simulink library "slrtnpcinverterlib"  (R2022b)
settings: Solver=VariableStepAuto  StartTime=0.0  StopTime=10.0  RelTol=1e-3
libraries: simulink x39, slrthdlutillib x6, $bdroot x3, hdlsllib x1
settings Model: Creator=chrisz  LastModifiedBy=chrisz
settings ModelReferenceCC: EnableRefExpFcnMdlSchedulingChecks=on

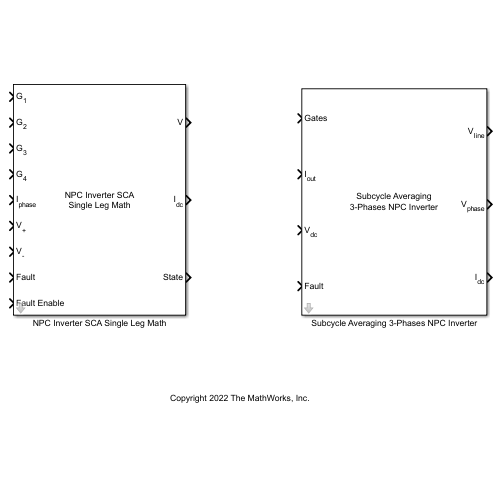
[thumbnail: Simulink's stored preview of the top-level diagram]
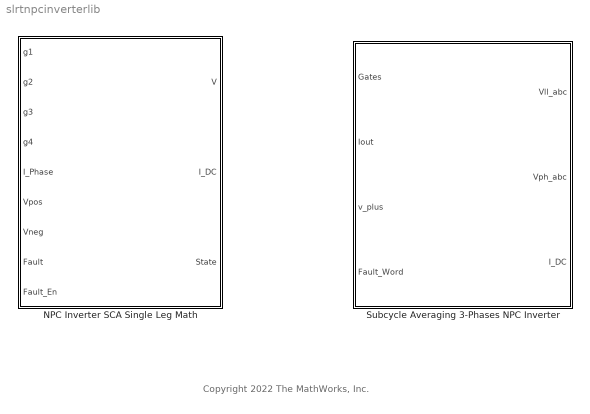
== system slrtnpcinverterlib ==
  note: Copyright 2022 The MathWorks, Inc.
  NPC Inverter SCA Single Leg Math : Subsystem  mask(NPC Inverter SCA Single Leg Math){rIGBT=0.1, vfIGBT=0.8, rDiode=0.2, vfDiode=0.6, rSnub=1e5, ts_Model=1e-6, ts_FPGA=5e-9}
      mask prompts: rIGBT "IGBT Resistance (Ohms):"; vfIGBT "IGBT Forward Voltage (V):"; rDiode "Diode Resistance (Ohms):"; vfDiode "Diode Forward Voltage (V):"; rSnub "Snubber resistance (Ohms):"; ts_Model "Model Time Step (s):"; ts_FPGA "FPGA Time Step (s):"
      mask help: This block implements the algorithm for a single leg of subcycle averaging NPC inverter. This model simulates FPGA clock level operations and is not suited for desktop simulation other than for validating the real-time model is accurate. It should primarily be used when generating HDL for real-time systems. Use standard blocks for desktop simulation.
      mask DialogControl Container6 Prompt: Simulation Parameters
      mask Display:
      | disp('NPC Inverter SCA\nSingle Leg Math');
      | 
      | port_label('input', 1, 'G_1','texmode','on');
      | port_label('input', 2, 'G_2','texmode','on');
      | port_label('input', 3, 'G_3','texmode','on');
      | port_label('input', 4, 'G_4','texmode','on');
      | port_label('input', 5, 'I_p_h_a_s_e','texmode','on');
      | port_label('input', 6, 'V_+','texmode','on');
      | port_label('input', 7, 'V_-','texmode','on');
      | port_label('input', 8, 'Fault');
      | port_label('input', 9, 'Fault Enable');
      | port_label('output', 1, 'V');
      | port_label('output', 2, 'I_d_c','texmode','on');
      | port_label('output', 3, 'State');
  Subcycle Averaging 3-Phases NPC Inverter : Subsystem  mask(Subcycle Averaging 3-Phases NPC Inverter){rIGBT=0.1, vfIGBT=0.8, rDiode=0.2, vfDiode=0.6, rSnub=1e5, ts_Model=1e-6, ts_FPGA=5e-9}
      mask prompts: rIGBT "IGBT Resistance (Ohms):"; vfIGBT "IGBT Forward Voltage (V):"; rDiode "Diode Resistance (Ohms):"; vfDiode "Diode Forward Voltage (V):"; rSnub "Snubber resistance (Ohms):"; ts_Model "Model Time Step (s):"; ts_FPGA "FPGA Time Step (s):"
      mask help:
      | HDL compatible implementation of subcycle averaging 3-phases NPC inverter. This model simulates FPGA clock level operations and is not suited for desktop simulation other than for validating the real-time model is accurate. It should primarily be used when generating HDL for real-time systems. Use standard blocks for desktop simulation.
      |
      | Model time step should be 1/10 of switching frequency to capture accurate switching waveforms. FPGA time step should be the fastest time step you can run your HIL FPGA at.
      mask DialogControl Container3 Prompt: Simulation Parameters
      mask Display:
      | disp('Subcycle Averaging\n3-Phases NPC Inverter')
      | port_label('input',1,'Gates');
      | port_label('input',2,'I_o_u_t','texmode','on');
      | port_label('input',3,'V_d_c','texmode','on');
      | port_label('input',4,'Fault');
      | 
      | port_label('output',1,'V_l_i_n_e','texmode','on');
      | port_label('output',2,'V_p_h_a_s_e','texmode','on');
      | port_label('output',3,'I_d_c','texmode','on');

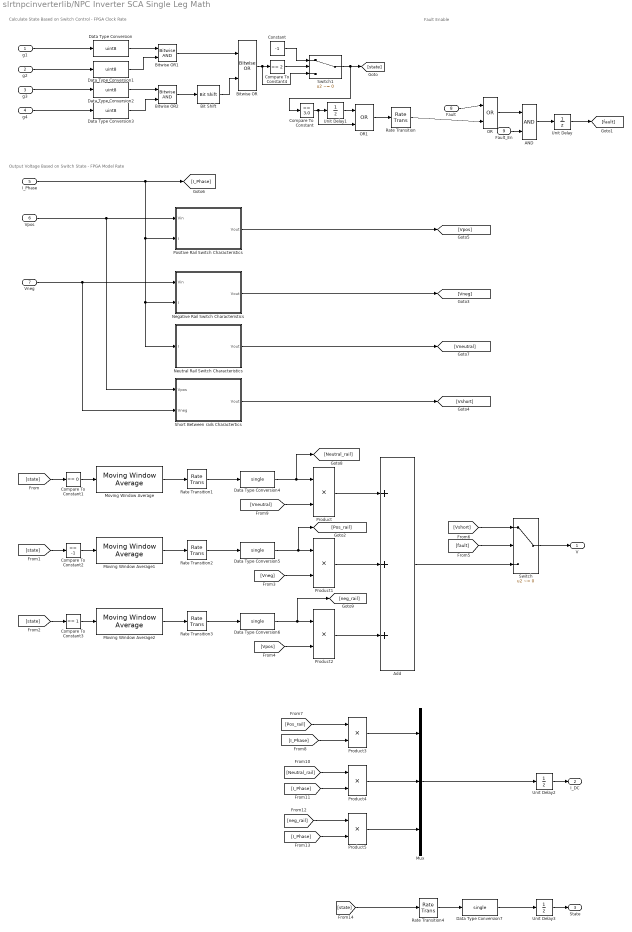
== system slrtnpcinverterlib/NPC Inverter SCA Single Leg Math ==
  note: Output Voltage Based on Switch State - FPGA Model Rate
  note: Fault Enable
  note: Calculate State Based on Switch Control - FPGA Clock Rate
  g1 : Inport
  g2 : Inport  Port=2
  g3 : Inport  Port=3
  g4 : Inport  Port=4
  I_Phase : Inport  Port=5
  Vpos : Inport  Port=6
  Vneg : Inport  Port=7
  Fault : Inport  Port=8
  Fault_En : Inport  Port=9
  AND : Logic  IconShape=distinctive  AllPortsSameDT=off  OutDataTypeStr=boolean
  Add : Sum  Inputs=+++
  Bit Shift : hdlsllib/Logic and Bit Operations/Bit Shift  mode=Shift Left Logical  N=1
  Bitwise OR : simulink/Logic and Bit Operations/Bitwise Operator  logicop=OR  UseBitMask=off  NumInputPorts=2  BitMask=bin2dec('11011001')  BitMaskRealWorld=Stored Integer
  Bitwise OR1 : simulink/Logic and Bit Operations/Bitwise Operator  logicop=AND  UseBitMask=off  NumInputPorts=2  BitMask=bin2dec('11011001')  BitMaskRealWorld=Stored Integer
  Bitwise OR2 : simulink/Logic and Bit Operations/Bitwise Operator  logicop=AND  UseBitMask=off  NumInputPorts=2  BitMask=bin2dec('11011001')  BitMaskRealWorld=Stored Integer
  Compare To Constant : simulink/Logic and Bit Operations/Compare To Constant  relop===  const=3.0  OutDataTypeStr=boolean
  Compare To Constant1 : simulink/Logic and Bit Operations/Compare To Constant  relop===  const=0  OutDataTypeStr=boolean
  Compare To Constant2 : simulink/Logic and Bit Operations/Compare To Constant  relop===  const=-1  OutDataTypeStr=boolean
  Compare To Constant3 : simulink/Logic and Bit Operations/Compare To Constant  relop===  const=1  OutDataTypeStr=boolean
  Compare To Constant4 : simulink/Logic and Bit Operations/Compare To Constant  relop===  const=2  OutDataTypeStr=boolean
  Constant : Constant  Value=-1  OutDataTypeStr=int8  SampleTime=-1
  Data Type Conversion{,1..3} (4 alike) : DataTypeConversion  OutDataTypeStr=uint8  SaturateOnIntegerOverflow=off  RndMeth=Floor
  Data Type Conversion{4..7} (4 alike) : DataTypeConversion  OutDataTypeStr=single  SaturateOnIntegerOverflow=off  RndMeth=Floor
  Moving Window Average : slrthdlutillib/Moving Window Average  sample_time=ts_FPGA  window_size=ts_Model
  Moving Window Average1 : slrthdlutillib/Moving Window Average  sample_time=ts_FPGA  window_size=ts_Model
  Moving Window Average2 : slrthdlutillib/Moving Window Average  sample_time=ts_FPGA  window_size=ts_Model
  Mux : Mux  Inputs=3
  Negative Rail Switch Characteristics : Subsystem
  Neutral Rail Switch Characteristics : Subsystem
  OR : Logic  Operator=OR  IconShape=distinctive  AllPortsSameDT=off  OutDataTypeStr=boolean
  OR1 : Logic  Operator=OR  IconShape=distinctive  AllPortsSameDT=off  OutDataTypeStr=boolean
  Positive Rail Switch Characteristics : Subsystem
  Product{,1..5} (6 alike) : Product
  Rate Transition{,1..4} (5 alike) : RateTransition  OutPortSampleTime=ts_Model
  Short Between rails Charactertics : Subsystem
  Switch : Switch  Criteria=u2 ~= 0  SaturateOnIntegerOverflow=off  InputSameDT=off
  Switch1 : Switch  Criteria=u2 ~= 0  OutDataTypeStr=int8  SaturateOnIntegerOverflow=off  InputSameDT=off
  Unit Delay{,1..3} (4 alike) : UnitDelay  SampleTime=-1  HasFrameUpgradeWarning=on
  V : Outport
  I_DC : Outport  Port=2
  State : Outport  Port=3
  wires:
  Fault/1 -> OR/1
  Data Type Conversion/1 -> Bitwise OR1/1
  Bitwise OR/1 -> Switch1/3, Compare To Constant4/1
  Data Type Conversion3/1 -> Bitwise OR2/2
  Data Type Conversion1/1 -> Bitwise OR1/2
  Data Type Conversion2/1 -> Bitwise OR2/1
  [state] -> Compare To Constant1/1
  g1/1 -> Data Type Conversion/1
  g2/1 -> Data Type Conversion1/1
  g3/1 -> Data Type Conversion2/1
  g4/1 -> Data Type Conversion3/1
  OR/1 -> AND/1
  Fault_En/1 -> AND/2
  AND/1 -> Unit Delay/1
  Unit Delay/1 -> [fault]
  Compare To Constant/1 -> OR1/2, Unit Delay1/1
  Unit Delay1/1 -> OR1/1
  Rate Transition/1 -> OR/2
  OR1/1 -> Rate Transition/1
  Vneg/1 -> Short Between rails Charactertics/2(Vneg), Negative Rail Switch Characteristics/1(Vin)
  Vpos/1 -> Short Between rails Charactertics/1(Vpos), Positive Rail Switch Characteristics/1(Vin)
  Positive Rail Switch Characteristics/1(Vout) -> [Vpos]
  Negative Rail Switch Characteristics/1(Vout) -> [Vneg]
  Short Between rails Charactertics/1(Vout) -> [Vshort]
  [state] -> Compare To Constant2/1
  [state] -> Compare To Constant3/1
  Compare To Constant1/1 -> Moving Window Average/1
  Compare To Constant2/1 -> Moving Window Average1/1
  Compare To Constant3/1 -> Moving Window Average2/1
  Moving Window Average/1 -> Rate Transition1/1
  Moving Window Average1/1 -> Rate Transition2/1
  Moving Window Average2/1 -> Rate Transition3/1
  Rate Transition1/1 -> Data Type Conversion4/1
  Rate Transition2/1 -> Data Type Conversion5/1
  Rate Transition3/1 -> Data Type Conversion6/1
  Data Type Conversion4/1 -> [Neutral_rail], Product/1
  [Vneutral] -> Product/2
  Data Type Conversion5/1 -> [Pos_rail], Product1/1
  [Vneg] -> Product1/2
  Data Type Conversion6/1 -> [neg_rail], Product2/1
  [Vpos] -> Product2/2
  Product/1 -> Add/1
  Product1/1 -> Add/2
  Product2/1 -> Add/3
  [fault] -> Switch/2
  [Vshort] -> Switch/1
  Add/1 -> Switch/3
  Switch/1 -> V/1
  [Pos_rail] -> Product3/1
  I_Phase/1 -> [I_Phase], Positive Rail Switch Characteristics/2(I), Neutral Rail Switch Characteristics/1(I), Negative Rail Switch Characteristics/2(I)
  [I_Phase] -> Product3/2
  Unit Delay2/1 -> I_DC/1
  Neutral Rail Switch Characteristics/1(Vout) -> [Vneutral]
  [Neutral_rail] -> Product4/1
  [I_Phase] -> Product4/2
  [neg_rail] -> Product5/1
  [I_Phase] -> Product5/2
  Product3/1 -> Mux/1
  Product4/1 -> Mux/2
  Product5/1 -> Mux/3
  Mux/1 -> Unit Delay2/1
  Bitwise OR2/1 -> Bit Shift/1
  Bit Shift/1 -> Bitwise OR/2
  Bitwise OR1/1 -> Bitwise OR/1
  Compare To Constant4/1 -> Switch1/2
  Switch1/1 -> Compare To Constant/1, [state]
  Constant/1 -> Switch1/1
  Data Type Conversion7/1 -> Unit Delay3/1
  Unit Delay3/1 -> State/1
  [state] -> Rate Transition4/1
  Rate Transition4/1 -> Data Type Conversion7/1

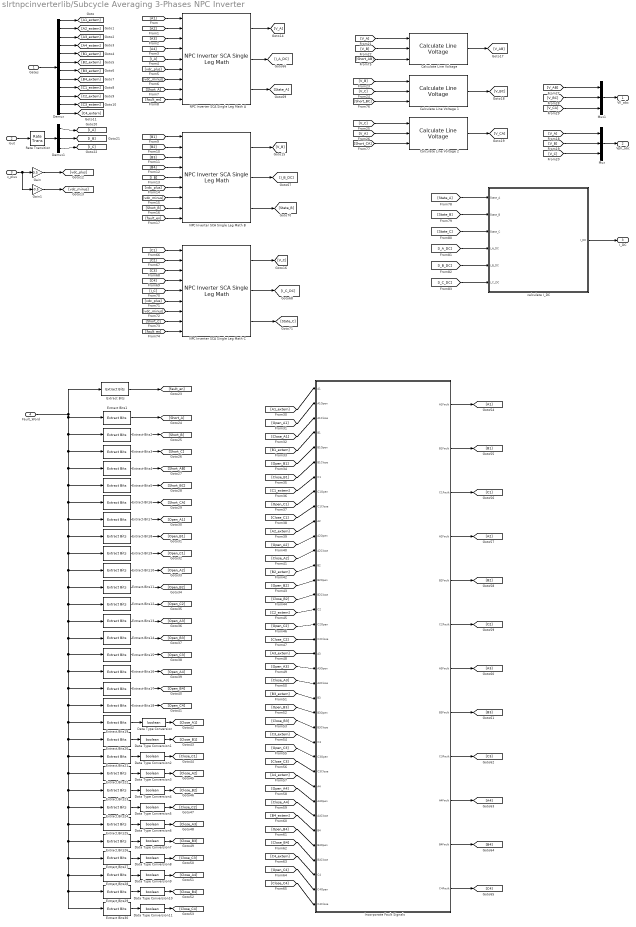
== system slrtnpcinverterlib/Subcycle Averaging 3-Phases NPC Inverter ==
  Gates : Inport
  Iout : Inport  Port=2
  v_plus : Inport  Port=3
  Fault_Word : Inport  Port=4
  "Calculate Line Voltage " : slrthdlutillib/Calculate Line Voltage 
  Calculate Line Voltage 1 : slrthdlutillib/Calculate Line Voltage 
  Calculate Line Voltage 2 : slrthdlutillib/Calculate Line Voltage 
  Data Type Conversion{,1..11} (12 alike) : DataTypeConversion  OutDataTypeStr=boolean  SaturateOnIntegerOverflow=off  RndMeth=Floor
  Demux : Demux  Outputs=12
  Demux1 : Demux  Outputs=3
  Extract Bits : simulink/Logic and Bit Operations/Extract Bits  bitsToExtract=Range of bits  numBits=8  bitIdxRange=31  outScalingMode=Treat bit field as an integer
  Extract Bits1 : simulink/Logic and Bit Operations/Extract Bits  bitsToExtract=Range of bits  numBits=8  bitIdxRange=0  outScalingMode=Treat bit field as an integer
  Extract Bits10 : simulink/Logic and Bit Operations/Extract Bits  bitsToExtract=Range of bits  numBits=8  bitIdxRange=9  outScalingMode=Treat bit field as an integer
  Extract Bits11 : simulink/Logic and Bit Operations/Extract Bits  bitsToExtract=Range of bits  numBits=8  bitIdxRange=10  outScalingMode=Treat bit field as an integer
  Extract Bits12 : simulink/Logic and Bit Operations/Extract Bits  bitsToExtract=Range of bits  numBits=8  bitIdxRange=11  outScalingMode=Treat bit field as an integer
  Extract Bits13 : simulink/Logic and Bit Operations/Extract Bits  bitsToExtract=Range of bits  numBits=8  bitIdxRange=12  outScalingMode=Treat bit field as an integer
  Extract Bits14 : simulink/Logic and Bit Operations/Extract Bits  bitsToExtract=Range of bits  numBits=8  bitIdxRange=13  outScalingMode=Treat bit field as an integer
  Extract Bits15 : simulink/Logic and Bit Operations/Extract Bits  bitsToExtract=Range of bits  numBits=8  bitIdxRange=14  outScalingMode=Treat bit field as an integer
  Extract Bits16 : simulink/Logic and Bit Operations/Extract Bits  bitsToExtract=Range of bits  numBits=8  bitIdxRange=15  outScalingMode=Treat bit field as an integer
  Extract Bits17 : simulink/Logic and Bit Operations/Extract Bits  bitsToExtract=Range of bits  numBits=8  bitIdxRange=16  outScalingMode=Treat bit field as an integer
  Extract Bits18 : simulink/Logic and Bit Operations/Extract Bits  bitsToExtract=Range of bits  numBits=8  bitIdxRange=17  outScalingMode=Treat bit field as an integer
  Extract Bits19 : simulink/Logic and Bit Operations/Extract Bits  bitsToExtract=Range of bits  numBits=8  bitIdxRange=18  outScalingMode=Treat bit field as an integer
  Extract Bits2 : simulink/Logic and Bit Operations/Extract Bits  bitsToExtract=Range of bits  numBits=8  bitIdxRange=1  outScalingMode=Treat bit field as an integer
  Extract Bits20 : simulink/Logic and Bit Operations/Extract Bits  bitsToExtract=Range of bits  numBits=8  bitIdxRange=19  outScalingMode=Treat bit field as an integer
  Extract Bits21 : simulink/Logic and Bit Operations/Extract Bits  bitsToExtract=Range of bits  numBits=8  bitIdxRange=20  outScalingMode=Treat bit field as an integer
  Extract Bits22 : simulink/Logic and Bit Operations/Extract Bits  bitsToExtract=Range of bits  numBits=8  bitIdxRange=21  outScalingMode=Treat bit field as an integer
  Extract Bits23 : simulink/Logic and Bit Operations/Extract Bits  bitsToExtract=Range of bits  numBits=8  bitIdxRange=22  outScalingMode=Treat bit field as an integer
  Extract Bits24 : simulink/Logic and Bit Operations/Extract Bits  bitsToExtract=Range of bits  numBits=8  bitIdxRange=23  outScalingMode=Treat bit field as an integer
  Extract Bits25 : simulink/Logic and Bit Operations/Extract Bits  bitsToExtract=Range of bits  numBits=8  bitIdxRange=24  outScalingMode=Treat bit field as an integer
  Extract Bits26 : simulink/Logic and Bit Operations/Extract Bits  bitsToExtract=Range of bits  numBits=8  bitIdxRange=25  outScalingMode=Treat bit field as an integer
  Extract Bits27 : simulink/Logic and Bit Operations/Extract Bits  bitsToExtract=Range of bits  numBits=8  bitIdxRange=26  outScalingMode=Treat bit field as an integer
  Extract Bits28 : simulink/Logic and Bit Operations/Extract Bits  bitsToExtract=Range of bits  numBits=8  bitIdxRange=27  outScalingMode=Treat bit field as an integer
  Extract Bits29 : simulink/Logic and Bit Operations/Extract Bits  bitsToExtract=Range of bits  numBits=8  bitIdxRange=28  outScalingMode=Treat bit field as an integer
  Extract Bits3 : simulink/Logic and Bit Operations/Extract Bits  bitsToExtract=Range of bits  numBits=8  bitIdxRange=2  outScalingMode=Treat bit field as an integer
  Extract Bits30 : simulink/Logic and Bit Operations/Extract Bits  bitsToExtract=Range of bits  numBits=8  bitIdxRange=29  outScalingMode=Treat bit field as an integer
  Extract Bits4 : simulink/Logic and Bit Operations/Extract Bits  bitsToExtract=Range of bits  numBits=8  bitIdxRange=3  outScalingMode=Treat bit field as an integer
  Extract Bits5 : simulink/Logic and Bit Operations/Extract Bits  bitsToExtract=Range of bits  numBits=8  bitIdxRange=4  outScalingMode=Treat bit field as an integer
  Extract Bits6 : simulink/Logic and Bit Operations/Extract Bits  bitsToExtract=Range of bits  numBits=8  bitIdxRange=5  outScalingMode=Treat bit field as an integer
  Extract Bits7 : simulink/Logic and Bit Operations/Extract Bits  bitsToExtract=Range of bits  numBits=8  bitIdxRange=6  outScalingMode=Treat bit field as an integer
  Extract Bits8 : simulink/Logic and Bit Operations/Extract Bits  bitsToExtract=Range of bits  numBits=8  bitIdxRange=7  outScalingMode=Treat bit field as an integer
  Extract Bits9 : simulink/Logic and Bit Operations/Extract Bits  bitsToExtract=Range of bits  numBits=8  bitIdxRange=8  outScalingMode=Treat bit field as an integer
  Gain : Gain  Gain=0.5
  Gain1 : Gain  Gain=-0.5
  Incorporate Fault Signals : Subsystem
  Mux : Mux  Inputs=3
  Mux1 : Mux  Inputs=3
  NPC Inverter SCA Single Leg Math A : $bdroot/NPC Inverter SCA Single Leg Math  rIGBT=rIGBT  vfIGBT=vfIGBT  rDiode=rDiode  vfDiode=vfDiode  rSnub=rSnub  ts_Model=ts_Model  ts_FPGA=ts_FPGA
  NPC Inverter SCA Single Leg Math B : $bdroot/NPC Inverter SCA Single Leg Math  rIGBT=rIGBT  vfIGBT=vfIGBT  rDiode=rDiode  vfDiode=vfDiode  rSnub=rSnub  ts_Model=ts_Model  ts_FPGA=ts_FPGA
  NPC Inverter SCA Single Leg Math C : $bdroot/NPC Inverter SCA Single Leg Math  rIGBT=rIGBT  vfIGBT=vfIGBT  rDiode=rDiode  vfDiode=vfDiode  rSnub=rSnub  ts_Model=ts_Model  ts_FPGA=ts_FPGA
  Rate Transition : RateTransition  OutPortSampleTime=ts_Model
  calculate I_DC : Subsystem
  Vll_abc : Outport
  Vph_abc : Outport  Port=2
  I_DC : Outport  Port=3
  wires:
  Gates/1 -> Demux/1
  Demux/1 -> [A1_extern]
  Demux/2 -> [A2_extern]
  Demux/3 -> [A3_extern]
  Demux/4 -> [A4_extern]
  Demux/5 -> [B1_extern]
  Demux/6 -> [B2_extern]
  Demux/7 -> [B3_extern]
  Demux/8 -> [B4_extern]
  Demux/9 -> [C1_extern]
  Demux/10 -> [C2_extern]
  Demux/11 -> [C3_extern]
  Demux/12 -> [C4_extern]
  Gain1/1 -> [vdc_minus]
  NPC Inverter SCA Single Leg Math A/1 -> [V_A]
  NPC Inverter SCA Single Leg Math B/1 -> [V_B]
  NPC Inverter SCA Single Leg Math C/1 -> [V_C]
  Mux/1 -> Vph_abc/1
  [V_A] -> Mux/1
  [V_B] -> Mux/2
  [V_C] -> Mux/3
  [V_A] -> "Calculate Line Voltage "/1
  [V_B] -> "Calculate Line Voltage "/2
  "Calculate Line Voltage "/1 -> [V_AB]
  [V_C] -> Calculate Line Voltage 1/2
  [V_B] -> Calculate Line Voltage 1/1
  Calculate Line Voltage 1/1 -> [V_BC]
  [V_A] -> Calculate Line Voltage 2/2
  [V_C] -> Calculate Line Voltage 2/1
  Calculate Line Voltage 2/1 -> [V_CA]
  Mux1/1 -> Vll_abc/1
  [V_AB] -> Mux1/1
  [V_BC] -> Mux1/2
  [V_CA] -> Mux1/3
  Demux1/1 -> [I_A]
  Demux1/2 -> [I_B]
  Demux1/3 -> [I_C]
  Fault_Word/1 -> Extract Bits/1, Extract Bits7/1, Extract Bits8/1, Extract Bits9/1, Extract Bits10/1, Extract Bits11/1, Extract Bits12/1, Extract Bits13/1, Extract Bits14/1, Extract Bits16/1, Extract Bits17/1, Extract Bits19/1, Extract Bits20/1, Extract Bits21/1, Extract Bits22/1, Extract Bits23/1, Extract Bits24/1, Extract Bits25/1, Extract Bits26/1, Extract Bits27/1, Extract Bits28/1, Extract Bits29/1, Extract Bits30/1, Extract Bits18/1, Extract Bits15/1, Extract Bits6/1, Extract Bits5/1, Extract Bits4/1, Extract Bits3/1, Extract Bits2/1, Extract Bits1/1
  Extract Bits/1 -> [fault_en]
  Extract Bits1/1 -> [Short_A]
  Extract Bits2/1 -> [Short_B]
  Extract Bits3/1 -> [Short_C]
  Extract Bits4/1 -> [Short_AB]
  Extract Bits5/1 -> [Short_BC]
  Extract Bits6/1 -> [Short_CA]
  Extract Bits7/1 -> [Open_A1]
  Extract Bits8/1 -> [Open_B1]
  Extract Bits9/1 -> [Open_C1]
  Extract Bits10/1 -> [Open_A2]
  Extract Bits12/1 -> [Open_C2]
  Extract Bits11/1 -> [Open_B2]
  Extract Bits13/1 -> [Open_A3]
  Extract Bits15/1 -> [Open_C3]
  Extract Bits14/1 -> [Open_B3]
  Extract Bits18/1 -> [Open_C4]
  Extract Bits17/1 -> [Open_B4]
  Extract Bits16/1 -> [Open_A4]
  [A1_extern] -> Incorporate Fault Signals/1(A1)
  [Open_A1] -> Incorporate Fault Signals/2(A1Open)
  [Close_A1] -> Incorporate Fault Signals/3(A1Close)
  [Close_B1] -> Incorporate Fault Signals/6(B1Close)
  [Open_B1] -> Incorporate Fault Signals/5(B1Open)
  [B1_extern] -> Incorporate Fault Signals/4(B1)
  [C1_extern] -> Incorporate Fault Signals/7(C1)
  [Open_C1] -> Incorporate Fault Signals/8(C1Open)
  [Close_C1] -> Incorporate Fault Signals/9(C1Close)
  [A2_extern] -> Incorporate Fault Signals/10(A2)
  [Open_A2] -> Incorporate Fault Signals/11(A2Open)
  [Close_A2] -> Incorporate Fault Signals/12(A2Close)
  [Close_B2] -> Incorporate Fault Signals/15(B2Close)
  [Open_B2] -> Incorporate Fault Signals/14(B2Open)
  [B2_extern] -> Incorporate Fault Signals/13(B2)
  [C2_extern] -> Incorporate Fault Signals/16(C2)
  [Open_C2] -> Incorporate Fault Signals/17(C2Open)
  [Close_C2] -> Incorporate Fault Signals/18(C2Close)
  [Close_A3] -> Incorporate Fault Signals/21(A3Close)
  [Open_A3] -> Incorporate Fault Signals/20(A3Open)
  [A3_extern] -> Incorporate Fault Signals/19(A3)
  [Close_B3] -> Incorporate Fault Signals/24(B3Close)
  [Open_B3] -> Incorporate Fault Signals/23(B3Open)
  [B3_extern] -> Incorporate Fault Signals/22(B3)
  [Close_C3] -> Incorporate Fault Signals/27(C3Close)
  [Open_C3] -> Incorporate Fault Signals/26(C3Open)
  [C3_extern] -> Incorporate Fault Signals/25(C3)
  [Close_A4] -> Incorporate Fault Signals/30(A4Close)
  [Open_A4] -> Incorporate Fault Signals/29(A4Open)
  [A4_extern] -> Incorporate Fault Signals/28(A4)
  [Close_B4] -> Incorporate Fault Signals/33(B4Close)
  [Open_B4] -> Incorporate Fault Signals/32(B4Open)
  [B4_extern] -> Incorporate Fault Signals/31(B4)
  [Close_C4] -> Incorporate Fault Signals/36(C4Close)
  [Open_C4] -> Incorporate Fault Signals/35(C4Open)
  [C4_extern] -> Incorporate Fault Signals/34(C4)
  Incorporate Fault Signals/1(A1Fault) -> [A1]
  Incorporate Fault Signals/2(B1Fault) -> [B1]
  Incorporate Fault Signals/3(C1Fault) -> [C1]
  Incorporate Fault Signals/4(A2Fault) -> [A2]
  Incorporate Fault Signals/5(B2Fault) -> [B2]
  Incorporate Fault Signals/6(C2Fault) -> [C2]
  Incorporate Fault Signals/7(A3Fault) -> [A3]
  Incorporate Fault Signals/8(B3Fault) -> [B3]
  Incorporate Fault Signals/9(C3Fault) -> [C3]
  Incorporate Fault Signals/10(A4Fault) -> [A4]
  Incorporate Fault Signals/11(B4Fault) -> [B4]
  Incorporate Fault Signals/12(C4Fault) -> [C4]
  [A1] -> NPC Inverter SCA Single Leg Math A/1
  [A2] -> NPC Inverter SCA Single Leg Math A/2
  [A3] -> NPC Inverter SCA Single Leg Math A/3
  [A4] -> NPC Inverter SCA Single Leg Math A/4
  [I_A] -> NPC Inverter SCA Single Leg Math A/5
  [vdc_plus] -> NPC Inverter SCA Single Leg Math A/6
  [vdc_minus] -> NPC Inverter SCA Single Leg Math A/7
  [Short_A] -> NPC Inverter SCA Single Leg Math A/8
  [fault_en] -> NPC Inverter SCA Single Leg Math A/9
  [B1] -> NPC Inverter SCA Single Leg Math B/1
  [B2] -> NPC Inverter SCA Single Leg Math B/2
  [B3] -> NPC Inverter SCA Single Leg Math B/3
  [B4] -> NPC Inverter SCA Single Leg Math B/4
  [I_B] -> NPC Inverter SCA Single Leg Math B/5
  [vdc_plus] -> NPC Inverter SCA Single Leg Math B/6
  [vdc_minus] -> NPC Inverter SCA Single Leg Math B/7
  [Short_B] -> NPC Inverter SCA Single Leg Math B/8
  [fault_en] -> NPC Inverter SCA Single Leg Math B/9
  [C1] -> NPC Inverter SCA Single Leg Math C/1
  [C2] -> NPC Inverter SCA Single Leg Math C/2
  [C3] -> NPC Inverter SCA Single Leg Math C/3
  [C4] -> NPC Inverter SCA Single Leg Math C/4
  [I_C] -> NPC Inverter SCA Single Leg Math C/5
  [vdc_plus] -> NPC Inverter SCA Single Leg Math C/6
  [vdc_minus] -> NPC Inverter SCA Single Leg Math C/7
  [Short_C] -> NPC Inverter SCA Single Leg Math C/8
  [fault_en] -> NPC Inverter SCA Single Leg Math C/9
  NPC Inverter SCA Single Leg Math A/2 -> [I_A_DC]
  NPC Inverter SCA Single Leg Math B/2 -> [I_B_DC]
  NPC Inverter SCA Single Leg Math C/2 -> [I_C_DC]
  [Short_AB] -> "Calculate Line Voltage "/3
  [Short_BC] -> Calculate Line Voltage 1/3
  [Short_CA] -> Calculate Line Voltage 2/3
  Data Type Conversion/1 -> [Close_A1]
  Extract Bits19/1 -> Data Type Conversion/1
  Data Type Conversion1/1 -> [Close_B1]
  Extract Bits20/1 -> Data Type Conversion1/1
  Extract Bits21/1 -> Data Type Conversion2/1
  Data Type Conversion2/1 -> [Close_C1]
  Extract Bits22/1 -> Data Type Conversion3/1
  Data Type Conversion3/1 -> [Close_A2]
  Extract Bits23/1 -> Data Type Conversion4/1
  Data Type Conversion4/1 -> [Close_B2]
  Extract Bits24/1 -> Data Type Conversion5/1
  Data Type Conversion5/1 -> [Close_C2]
  Extract Bits25/1 -> Data Type Conversion6/1
  Extract Bits26/1 -> Data Type Conversion7/1
  Extract Bits27/1 -> Data Type Conversion8/1
  Extract Bits28/1 -> Data Type Conversion9/1
  Extract Bits29/1 -> Data Type Conversion10/1
  Data Type Conversion6/1 -> [Close_A3]
  Data Type Conversion7/1 -> [Close_B3]
  Data Type Conversion8/1 -> [Close_C3]
  Data Type Conversion9/1 -> [Close_A4]
  Data Type Conversion10/1 -> [Close_B4]
  Extract Bits30/1 -> Data Type Conversion11/1
  Data Type Conversion11/1 -> [Close_C4]
  Iout/1 -> Rate Transition/1
  Rate Transition/1 -> Demux1/1
  v_plus/1 -> Gain1/1, Gain/1
  Gain/1 -> [vdc_plus]
  NPC Inverter SCA Single Leg Math A/3 -> [State_A]
  NPC Inverter SCA Single Leg Math B/3 -> [State_B]
  NPC Inverter SCA Single Leg Math C/3 -> [State_C]
  calculate I_DC/1(I_DC) -> I_DC/1
  [State_A] -> calculate I_DC/1(State_A)
  [State_B] -> calculate I_DC/2(State_B)
  [State_C] -> calculate I_DC/3(State_C)
  [I_A_DC] -> calculate I_DC/4(I_A_DC)
  [I_B_DC] -> calculate I_DC/5(I_B_DC)
  [I_C_DC] -> calculate I_DC/6(I_C_DC)

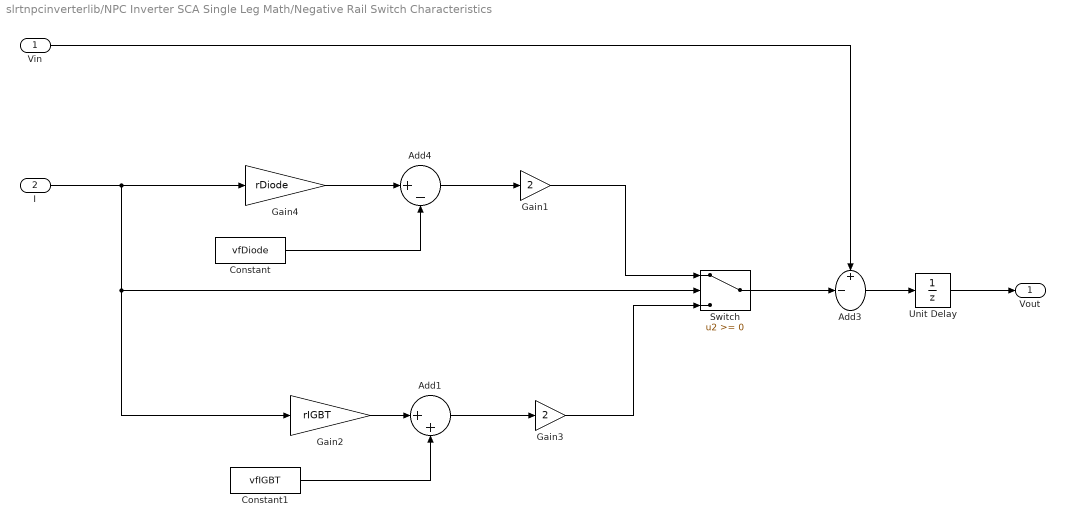
== system slrtnpcinverterlib/NPC Inverter SCA Single Leg Math/Negative Rail Switch Characteristics ==
  Vin : Inport
  I : Inport  Port=2
  Add1 : Sum  Inputs=|++
  Add3 : Sum  Inputs=+-|
  Add4 : Sum  Inputs=|+-
  Constant : Constant  Value=vfDiode  OutDataTypeStr=single  SampleTime=ts_Model
  Constant1 : Constant  Value=vfIGBT  OutDataTypeStr=single  SampleTime=ts_Model
  Gain1 : Gain  Gain=2
  Gain2 : Gain  Gain=rIGBT
  Gain3 : Gain  Gain=2
  Gain4 : Gain  Gain=rDiode
  Switch : Switch  SaturateOnIntegerOverflow=off  InputSameDT=off
  Unit Delay : UnitDelay  SampleTime=-1  HasFrameUpgradeWarning=on
  Vout : Outport
  wires:
  I/1 -> Gain2/1, Switch/2, Gain4/1
  Unit Delay/1 -> Vout/1
  Vin/1 -> Add3/1
  Add1/1 -> Gain3/1
  Constant1/1 -> Add1/2
  Gain2/1 -> Add1/1
  Gain3/1 -> Switch/3
  Gain4/1 -> Add4/1
  Constant/1 -> Add4/2
  Add4/1 -> Gain1/1
  Add3/1 -> Unit Delay/1
  Switch/1 -> Add3/2
  Gain1/1 -> Switch/1

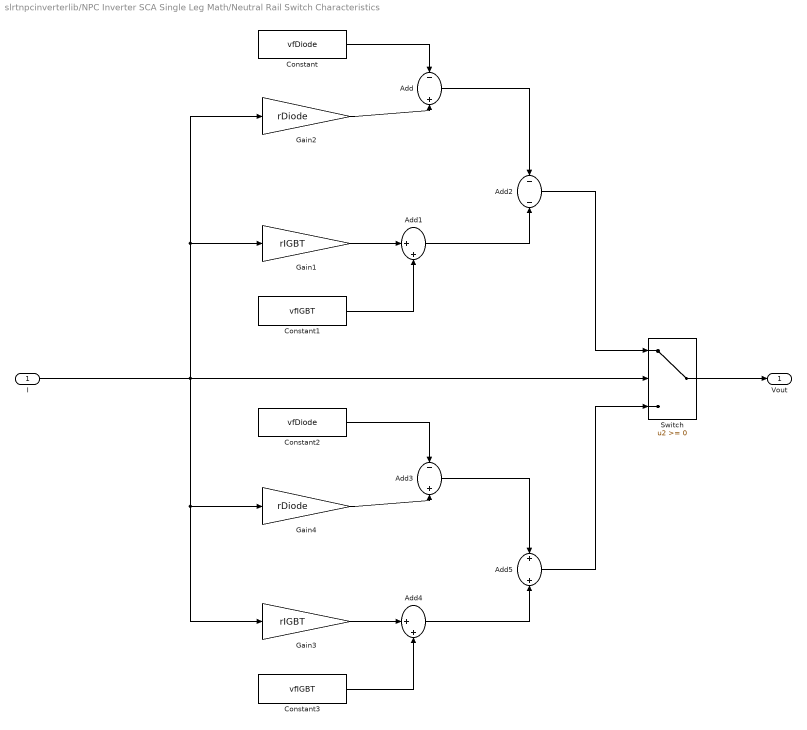
== system slrtnpcinverterlib/NPC Inverter SCA Single Leg Math/Neutral Rail Switch Characteristics ==
  I : Inport
  Add : Sum  Inputs=-+
  Add1 : Sum  Inputs=|++
  Add2 : Sum  Inputs=--
  Add3 : Sum  Inputs=-+
  Add4 : Sum  Inputs=|++
  Add5 : Sum
  Constant : Constant  Value=vfDiode  OutDataTypeStr=single  SampleTime=ts_Model
  Constant1 : Constant  Value=vfIGBT  OutDataTypeStr=single  SampleTime=ts_Model
  Constant2 : Constant  Value=vfDiode  OutDataTypeStr=single  SampleTime=ts_Model
  Constant3 : Constant  Value=vfIGBT  OutDataTypeStr=single  SampleTime=ts_Model
  Gain1 : Gain  Gain=rIGBT
  Gain2 : Gain  Gain=rDiode
  Gain3 : Gain  Gain=rIGBT
  Gain4 : Gain  Gain=rDiode
  Switch : Switch  SaturateOnIntegerOverflow=off  InputSameDT=off
  Vout : Outport
  wires:
  Gain1/1 -> Add1/1
  Constant1/1 -> Add1/2
  Add1/1 -> Add2/2
  Add5/1 -> Switch/3
  Add2/1 -> Switch/1
  Switch/1 -> Vout/1
  I/1 -> Gain4/1, Gain3/1, Gain2/1, Gain1/1, Switch/2
  Gain3/1 -> Add4/1
  Add4/1 -> Add5/2
  Constant3/1 -> Add4/2
  Gain2/1 -> Add/2
  Constant/1 -> Add/1
  Add/1 -> Add2/1
  Gain4/1 -> Add3/2
  Constant2/1 -> Add3/1
  Add3/1 -> Add5/1

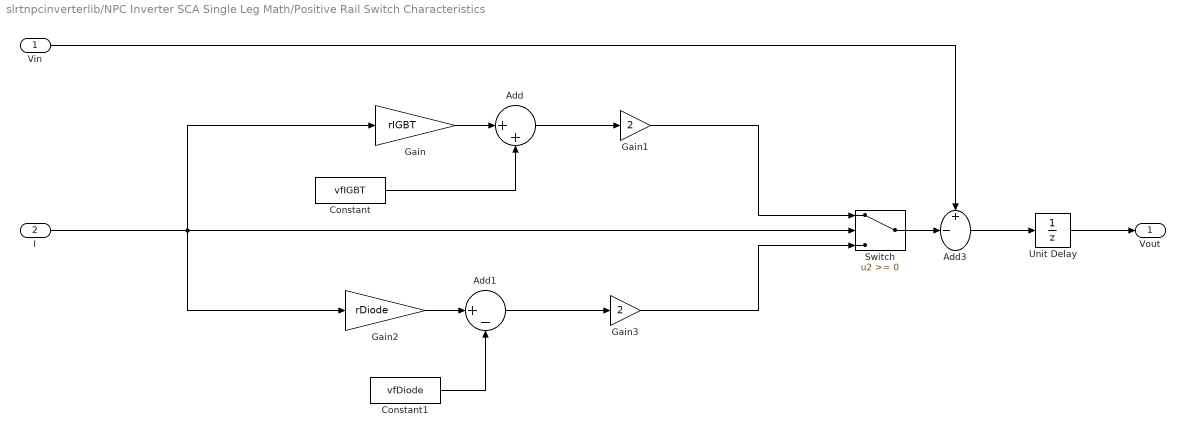
== system slrtnpcinverterlib/NPC Inverter SCA Single Leg Math/Positive Rail Switch Characteristics ==
  Vin : Inport
  I : Inport  Port=2
  Add : Sum  Inputs=|++
  Add1 : Sum  Inputs=|+-
  Add3 : Sum  Inputs=+-|
  Constant : Constant  Value=vfIGBT  OutDataTypeStr=single  SampleTime=ts_Model
  Constant1 : Constant  Value=vfDiode  OutDataTypeStr=single  SampleTime=ts_Model
  Gain : Gain  Gain=rIGBT
  Gain1 : Gain  Gain=2
  Gain2 : Gain  Gain=rDiode
  Gain3 : Gain  Gain=2
  Switch : Switch  SaturateOnIntegerOverflow=off  InputSameDT=off
  Unit Delay : UnitDelay  SampleTime=-1  HasFrameUpgradeWarning=on
  Vout : Outport
  wires:
  I/1 -> Gain2/1, Switch/2, Gain/1
  Gain/1 -> Add/1
  Constant/1 -> Add/2
  Add/1 -> Gain1/1
  Unit Delay/1 -> Vout/1
  Vin/1 -> Add3/1
  Gain3/1 -> Switch/3
  Gain2/1 -> Add1/1
  Add1/1 -> Gain3/1
  Constant1/1 -> Add1/2
  Add3/1 -> Unit Delay/1
  Switch/1 -> Add3/2
  Gain1/1 -> Switch/1

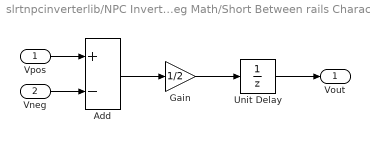
== system slrtnpcinverterlib/NPC Inverter SCA Single Leg Math/Short Between rails Charactertics ==
  Vpos : Inport
  Vneg : Inport  Port=2
  Add : Sum  Inputs=+-
  Gain : Gain  Gain=1/2
  Unit Delay : UnitDelay  SampleTime=-1  HasFrameUpgradeWarning=on
  Vout : Outport
  wires:
  Vpos/1 -> Add/1
  Vneg/1 -> Add/2
  Add/1 -> Gain/1
  Gain/1 -> Unit Delay/1
  Unit Delay/1 -> Vout/1

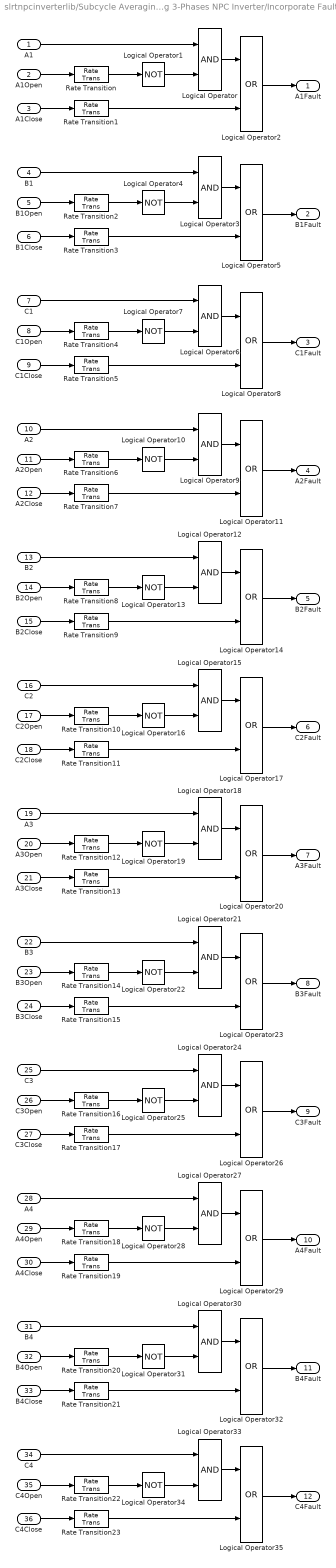
== system slrtnpcinverterlib/Subcycle Averaging 3-Phases NPC Inverter/Incorporate Fault Signals ==
  A1 : Inport
  A1Open : Inport  Port=2
  A1Close : Inport  Port=3
  B1 : Inport  Port=4
  B1Open : Inport  Port=5
  B1Close : Inport  Port=6
  C1 : Inport  Port=7
  C1Open : Inport  Port=8
  C1Close : Inport  Port=9
  A2 : Inport  Port=10
  A2Open : Inport  Port=11
  A2Close : Inport  Port=12
  B2 : Inport  Port=13
  B2Open : Inport  Port=14
  B2Close : Inport  Port=15
  C2 : Inport  Port=16
  C2Open : Inport  Port=17
  C2Close : Inport  Port=18
  A3 : Inport  Port=19
  A3Open : Inport  Port=20
  A3Close : Inport  Port=21
  B3 : Inport  Port=22
  B3Open : Inport  Port=23
  B3Close : Inport  Port=24
  C3 : Inport  Port=25
  C3Open : Inport  Port=26
  C3Close : Inport  Port=27
  A4 : Inport  Port=28
  A4Open : Inport  Port=29
  A4Close : Inport  Port=30
  B4 : Inport  Port=31
  B4Open : Inport  Port=32
  B4Close : Inport  Port=33
  C4 : Inport  Port=34
  C4Open : Inport  Port=35
  C4Close : Inport  Port=36
  Logical Operator{,3,6,9,12,15,18,21,24,27,30,33} (12 alike) : Logic  AllPortsSameDT=off  OutDataTypeStr=boolean
  Logical Operator{1,4,7,10,13,16,19,22,25,28,31,34} (12 alike) : Logic  Operator=NOT  AllPortsSameDT=off  OutDataTypeStr=boolean
  Logical Operator{2,5,8,11,14,17,20,23,26,29,32,35} (12 alike) : Logic  Operator=OR  AllPortsSameDT=off  OutDataTypeStr=boolean
  Rate Transition{,1..23} (24 alike) : RateTransition
  A1Fault : Outport
  B1Fault : Outport  Port=2
  C1Fault : Outport  Port=3
  A2Fault : Outport  Port=4
  B2Fault : Outport  Port=5
  C2Fault : Outport  Port=6
  A3Fault : Outport  Port=7
  B3Fault : Outport  Port=8
  C3Fault : Outport  Port=9
  A4Fault : Outport  Port=10
  B4Fault : Outport  Port=11
  C4Fault : Outport  Port=12
  wires:
  A1Open/1 -> Rate Transition/1
  A1Close/1 -> Rate Transition1/1
  Rate Transition/1 -> Logical Operator1/1
  Logical Operator1/1 -> Logical Operator/2
  A1/1 -> Logical Operator/1
  Logical Operator/1 -> Logical Operator2/1
  Rate Transition1/1 -> Logical Operator2/2
  Logical Operator2/1 -> A1Fault/1
  Rate Transition3/1 -> Logical Operator5/2
  B1Close/1 -> Rate Transition3/1
  Logical Operator4/1 -> Logical Operator3/2
  Rate Transition2/1 -> Logical Operator4/1
  B1/1 -> Logical Operator3/1
  Logical Operator5/1 -> B1Fault/1
  Logical Operator3/1 -> Logical Operator5/1
  B1Open/1 -> Rate Transition2/1
  Rate Transition5/1 -> Logical Operator8/2
  C1Close/1 -> Rate Transition5/1
  Logical Operator7/1 -> Logical Operator6/2
  Rate Transition4/1 -> Logical Operator7/1
  C1/1 -> Logical Operator6/1
  Logical Operator8/1 -> C1Fault/1
  Logical Operator6/1 -> Logical Operator8/1
  C1Open/1 -> Rate Transition4/1
  Rate Transition7/1 -> Logical Operator11/2
  A2Close/1 -> Rate Transition7/1
  Logical Operator10/1 -> Logical Operator9/2
  Rate Transition6/1 -> Logical Operator10/1
  Logical Operator15/1 -> Logical Operator17/1
  Rate Transition10/1 -> Logical Operator16/1
  C2/1 -> Logical Operator15/1
  Logical Operator16/1 -> Logical Operator15/2
  Logical Operator17/1 -> C2Fault/1
  Rate Transition11/1 -> Logical Operator17/2
  Rate Transition9/1 -> Logical Operator14/2
  A2/1 -> Logical Operator9/1
  Logical Operator11/1 -> A2Fault/1
  B2/1 -> Logical Operator12/1
  Logical Operator12/1 -> Logical Operator14/1
  C2Close/1 -> Rate Transition11/1
  C2Open/1 -> Rate Transition10/1
  B2Close/1 -> Rate Transition9/1
  Logical Operator13/1 -> Logical Operator12/2
  Logical Operator14/1 -> B2Fault/1
  B2Open/1 -> Rate Transition8/1
  Rate Transition8/1 -> Logical Operator13/1
  Logical Operator9/1 -> Logical Operator11/1
  A2Open/1 -> Rate Transition6/1
  Rate Transition13/1 -> Logical Operator20/2
  A3Close/1 -> Rate Transition13/1
  Logical Operator19/1 -> Logical Operator18/2
  Rate Transition12/1 -> Logical Operator19/1
  Logical Operator24/1 -> Logical Operator26/1
  Rate Transition16/1 -> Logical Operator25/1
  C3/1 -> Logical Operator24/1
  Logical Operator25/1 -> Logical Operator24/2
  Logical Operator26/1 -> C3Fault/1
  Rate Transition17/1 -> Logical Operator26/2
  Rate Transition15/1 -> Logical Operator23/2
  A3/1 -> Logical Operator18/1
  Logical Operator20/1 -> A3Fault/1
  B3/1 -> Logical Operator21/1
  Logical Operator21/1 -> Logical Operator23/1
  C3Close/1 -> Rate Transition17/1
  C3Open/1 -> Rate Transition16/1
  B3Close/1 -> Rate Transition15/1
  Logical Operator22/1 -> Logical Operator21/2
  Logical Operator23/1 -> B3Fault/1
  B3Open/1 -> Rate Transition14/1
  Rate Transition14/1 -> Logical Operator22/1
  Logical Operator18/1 -> Logical Operator20/1
  A3Open/1 -> Rate Transition12/1
  Rate Transition19/1 -> Logical Operator29/2
  A4Close/1 -> Rate Transition19/1
  Logical Operator28/1 -> Logical Operator27/2
  Rate Transition18/1 -> Logical Operator28/1
  Logical Operator33/1 -> Logical Operator35/1
  Rate Transition22/1 -> Logical Operator34/1
  C4/1 -> Logical Operator33/1
  Logical Operator34/1 -> Logical Operator33/2
  Logical Operator35/1 -> C4Fault/1
  Rate Transition23/1 -> Logical Operator35/2
  Rate Transition21/1 -> Logical Operator32/2
  A4/1 -> Logical Operator27/1
  Logical Operator29/1 -> A4Fault/1
  B4/1 -> Logical Operator30/1
  Logical Operator30/1 -> Logical Operator32/1
  C4Close/1 -> Rate Transition23/1
  C4Open/1 -> Rate Transition22/1
  B4Close/1 -> Rate Transition21/1
  Logical Operator31/1 -> Logical Operator30/2
  Logical Operator32/1 -> B4Fault/1
  B4Open/1 -> Rate Transition20/1
  Rate Transition20/1 -> Logical Operator31/1
  Logical Operator27/1 -> Logical Operator29/1
  A4Open/1 -> Rate Transition18/1

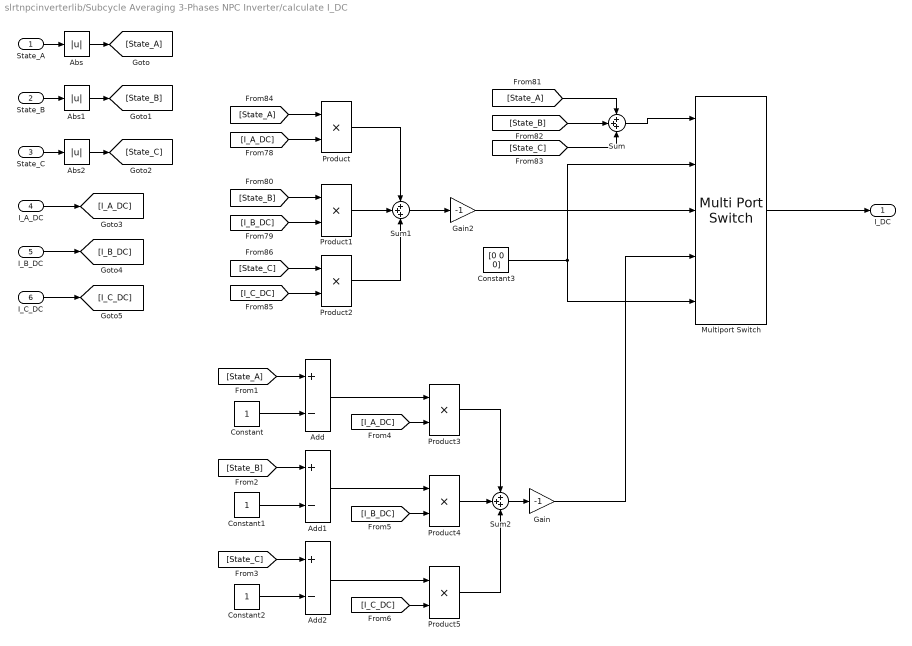
== system slrtnpcinverterlib/Subcycle Averaging 3-Phases NPC Inverter/calculate I_DC ==
  State_A : Inport
  State_B : Inport  Port=2
  State_C : Inport  Port=3
  I_A_DC : Inport  Port=4
  I_B_DC : Inport  Port=5
  I_C_DC : Inport  Port=6
  Abs : Abs  SaturateOnIntegerOverflow=off
  Abs1 : Abs  SaturateOnIntegerOverflow=off
  Abs2 : Abs  SaturateOnIntegerOverflow=off
  Add : Sum  Inputs=+-
  Add1 : Sum  Inputs=+-
  Add2 : Sum  Inputs=+-
  Constant : Constant  OutDataTypeStr=single  SampleTime=ts_Model
  Constant1 : Constant  OutDataTypeStr=single  SampleTime=ts_Model
  Constant2 : Constant  OutDataTypeStr=single  SampleTime=ts_Model
  Constant3 : Constant  Value=[0 0 0]  OutDataTypeStr=single  SampleTime=ts_Model
  Gain : Gain  Gain=-1
  Gain2 : Gain  Gain=-1
  Multiport Switch : MultiPortSwitch  DataPortOrder=Zero-based contiguous  Inputs=4  zeroidx=on  SaturateOnIntegerOverflow=off  InputSameDT=off
  Product{,1..5} (6 alike) : Product
  Sum : Sum  Inputs=+++
  Sum1 : Sum  Inputs=+++
  Sum2 : Sum  Inputs=+++
  I_DC : Outport
  wires:
  Product/1 -> Sum1/1
  [State_A] -> Product/1
  [I_A_DC] -> Product/2
  [State_B] -> Product1/1
  [I_C_DC] -> Product2/2
  Sum1/1 -> Gain2/1
  [I_B_DC] -> Product1/2
  [State_C] -> Product2/1
  Multiport Switch/1 -> I_DC/1
  [State_C] -> Sum/3
  Product1/1 -> Sum1/2
  [State_A] -> Sum/1
  Gain2/1 -> Multiport Switch/3
  [State_B] -> Sum/2
  Product2/1 -> Sum1/3
  Sum/1 -> Multiport Switch/1
  I_A_DC/1 -> [I_A_DC]
  I_B_DC/1 -> [I_B_DC]
  I_C_DC/1 -> [I_C_DC]
  [State_A] -> Add/1
  Constant/1 -> Add/2
  [State_B] -> Add1/1
  Constant1/1 -> Add1/2
  [State_C] -> Add2/1
  Constant2/1 -> Add2/2
  Add/1 -> Product3/1
  [I_A_DC] -> Product3/2
  [I_B_DC] -> Product4/2
  Add1/1 -> Product4/1
  [I_C_DC] -> Product5/2
  Add2/1 -> Product5/1
  Product3/1 -> Sum2/1
  Product4/1 -> Sum2/2
  Product5/1 -> Sum2/3
  Sum2/1 -> Gain/1
  Gain/1 -> Multiport Switch/4
  Constant3/1 -> Multiport Switch/5, Multiport Switch/2
  State_A/1 -> Abs/1
  Abs/1 -> [State_A]
  State_B/1 -> Abs1/1
  Abs1/1 -> [State_B]
  Abs2/1 -> [State_C]
  State_C/1 -> Abs2/1
